simulink model "validation"  (R2020a)
settings: Solver=VariableStepAuto  StartTime=0.0  StopTime=0.5  RelTol=1e-3
undefined symbols (not defined in the file): Te, Z0, Z00, Z1, Z11
settings Model: Creator=housni  LastModifiedBy=housni

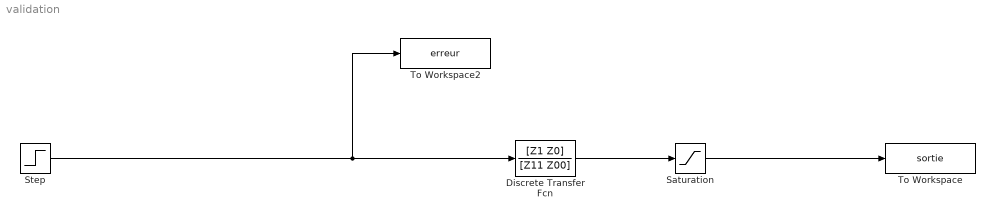
== system validation ==
  Discrete Transfer Fcn : DiscreteTransferFcn  Numerator=[Z1 Z0]  Denominator=[Z11 Z00]  SampleTime=Te
  Saturation : Saturate
  Step : Step  Time=0.01  After=0.1  SampleTime=0
  To Workspace : ToWorkspace  VariableName=sortie  SaveFormat=Timeseries  SampleTime=-1
  To Workspace2 : ToWorkspace  VariableName=erreur  SaveFormat=Timeseries  SampleTime=-1
  wires:
  Step/1 -> Discrete Transfer Fcn/1, To Workspace2/1
  Discrete Transfer Fcn/1 -> Saturation/1
  Saturation/1 -> To Workspace/1
